simulink model "pmsmctrl"  (R2018a)
settings: Solver=FixedStepDiscrete  StartTime=0.0  StopTime=10.0  FixedStep=FastTsample / 10.  RelTol=1e-3  EnableMultiTasking=on
model workspace (MATLAB code in the model file):
  | cmdLim = Simulink.Parameter;
  | cmdLim.Value = 15;
  | cmdLim.Description = 'Limit for controlling the maximum surface command angle.';
  | cmdLim.Min = 0;
  | cmdLim.Max = 90;
  | cmdLim.DocUnits = 'deg';
  | 
  | dispGain = Simulink.Parameter;
  | dispGain.Value = 0.75;
  | dispGain.Description = 'Gain applied to the displacement error.';
  | dispGain.Min = 0;
  | dispGain.Max = [];
  | dispGain.DocUnits = 'deg/sec/deg';
  | 
  | dispLim = Simulink.Parameter;
  | dispLim.Value = 30;
  | dispLim.Description = 'Limit for controlling the maximum commanded angle.';
  | dispLim.Min = 0;
  | dispLim.Max = 180;
  | dispLim.DocUnits = 'deg';
  | 
  | intGain = Simulink.Parameter;
  | intGain.Value = 0.5;
  | intGain.Description = 'Gain applied to the integral error.';
  | intGain.Min = 0;
  | intGain.Max = [];
  | intGain.DocUnits = 'deg/sec/deg/sec';
  | 
  | intLim = Simulink.Parameter;
  | intLim.Value = 5;
  | intLim.Description = 'Limit for controlling the maximum commanded angle.';
  | intLim.Min = 0;
  | intLim.Max = 90;
  | intLim.DocUnits = 'deg';
  | 
  | rateGain = Simulink.Parameter;
  | rateGain.Value = 2;
  | rateGain.Description = 'Gain applied to the rate error.';
  | rateGain.Min = 0;
  | rateGain.Max = [];
  | rateGain.DocUnits = 'deg/deg/sec';
  | 
  | rateLim = Simulink.Parameter;
  | rateLim.Value = 6;
  | rateLim.Description = 'Limit for controlling the maximum commanded angle.';
  | rateLim.Min = 0;
  | rateLim.Max = 180;
  | rateLim.DocUnits = 'deg/sec';
  | 
  | hdgGain = Simulink.Parameter;
  | hdgGain.Value = 0.015;
undefined symbols (not defined in the file): MtrParams
libraries: powerlib_meascontrol x1
settings Model: RequirementInfo={} %GIDa_fe9045fd_0412_4b6e_8206_617cc20e6fde  FPTRunName=Active  Creator=elrobotista  LastModifiedBy=elrobotista
settings SolverCC: MinimalZcImpactIntegration=on
settings DataIOCC: SaveFormat=StructureWithTime  SaveOutput=off  SignalLogging=off  DSMLogging=off  SaveTime=off
settings OptimizationCC: DefaultParameterBehavior=Inlined  UseDivisionForNetSlopeComputation=on  UseFloatMulNetSlope=on  DefaultUnderspecifiedDataType=single  UseSpecifiedMinMax=on  InlineInvariantSignals=on  EnhancedBackFolding=on  PassReuseOutputArgsAs=Individual arguments  ZeroExternalMemoryAtStartup=off  ZeroInternalMemoryAtStartup=off  NoFixptDivByZeroProtection=on  EfficientFloat2IntCast=on  LifeSpan=1  OptimizeBlockOrder=speed  DifferentSizesBufferReuse=on  OptimizationCustomize=off  LabelGuidedReuse=on
settings DebuggingCC: AllowSymbolicDim=off  StrictBusMsg=ErrorOnBusTreatedAsVector  SFUnexpectedBacktrackingDiag=warning  SFNoUnconditionalDefaultTransitionDiag=warning  SFExecutionAtInitializationDiag=none
settings HardwareCC: ProdBitPerPointer=32  ProdBitPerSizeT=32  ProdBitPerPtrDiffT=32  ProdLargestAtomicInteger=Long  ProdLargestAtomicFloat=Double  ProdWordSize=32  ProdHWDeviceType=ARM Compatible->ARM Cortex
settings SFSimCC: MATLABDynamicMemAlloc=off
settings RTWCC: SystemTargetFile=ert.tlc  GenCodeOnly=on  PackageGeneratedCodeAndArtifacts=on  TemplateMakefile=ert_default_tmf  GenerateReport=on  BuildConfiguration=Faster Runs  IncludeHyperlinkInReport=on  LaunchReport=on  GenerateTraceInfo=on  GenerateTraceReport=on  GenerateTraceReportSl=on  GenerateTraceReportSf=on  GenerateTraceReportEml=on  GenerateCodeMetricsReport=on
settings CodeAppCC: ForceParamTrailComments=on  IgnoreCustomStorageClasses=off  OperatorAnnotations=on  SimulinkDataObjDesc=on  SFDataObjDesc=on  CustomSymbolStrGlobalVar=rt$N$M  CustomSymbolStrType=$N$M  CustomSymbolStrFcn=$N$M$F  CustomSymbolStrMacro=$N$M  InsertBlockDesc=on  EnableCustomComments=on  ReqsInCode=on
settings ERTTargetCC: TargetLangStandard=C99 (ISO)  MultiwordLength=2048  GenerateFullHeader=off  IncludeMdlTerminateFcn=off  SuppressErrorStatus=on  ERTCustomFileBanners=off  SupportAbsoluteTime=off  MultiInstanceERTCode=on  CodeInterfacePackaging=Reusable function  SupportNonFinite=off  SupportComplex=off  RemoveDisableFunc=on  InlinedParameterPlacement=NonHierarchical  MultiInstanceErrorCode=Warning  ERTCustomFileTemplate=example_file_process.tlc  ERTFilePackagingFormat=CompactWithDataFile
settings ConfigComp: CovScope=ReferencedModels  CovSaveName=covdata_rollAP  CovMetricSettings=dcmtrwe  CovHTMLOptions=-sRT=1 -aTS=1 -bRG=1 -bTC=1 -hTR=1 -nFC=0 -scm=1 -bcm=1 -xEv=0  CovSaveCumulativeToWorkspaceVar=on  CovSaveSingleToWorkspaceVar=on  CovCumulativeVarName=covCumulativeData_rollAP  CovReportOnPause=off  CovExternalEMLEnable=off  CovSFcnEnable=off

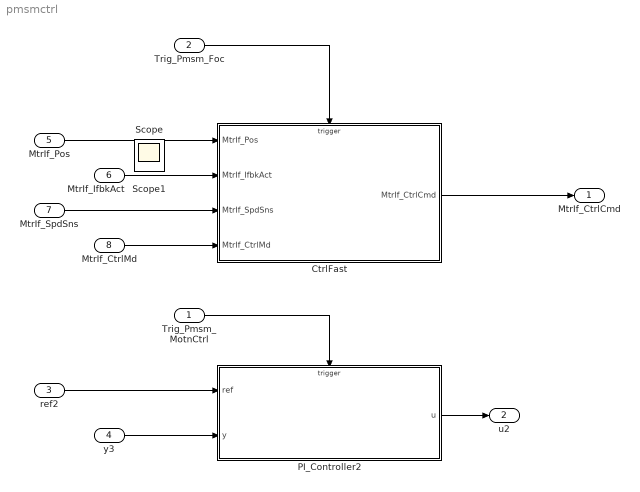
== system pmsmctrl ==
  Trig_Pmsm_MotnCtrl : Inport  OutDataTypeStr=double  OutputFunctionCall=on
  Trig_Pmsm_Foc : Inport  Port=2  OutDataTypeStr=double  OutputFunctionCall=on
  ref2 : Inport  Port=3
  y3 : Inport  Port=4
  MtrIf_Pos : Inport  Port=5
  MtrIf_IfbkAct : Inport  Port=6  PortDimensions=3
  MtrIf_SpdSns : Inport  Port=7
  MtrIf_CtrlMd : Inport  Port=8  OutDataTypeStr=Enum: MtrCtrlMd
  CtrlFast : Subsystem  TreatAsAtomicUnit=on  RTWFcnName=foo
  PI_Controller2 : Subsystem  TreatAsAtomicUnit=on  RTWFcnName=foo
  MtrIf_CtrlCmd : Outport
  u2 : Outport  Port=2
  Scope : Scope
  Scope1 : Scope
  wires:
  Trig_Pmsm_Foc/1 -> CtrlFast/Trigger
  Trig_Pmsm_MotnCtrl/1 -> PI_Controller2/Trigger
  PI_Controller2/1(u) -> u2/1
  ref2/1 -> PI_Controller2/1(ref)
  y3/1 -> PI_Controller2/2(y)
  MtrIf_Pos/1 -> CtrlFast/1(MtrIf_Pos)
  MtrIf_IfbkAct/1 -> CtrlFast/2(MtrIf_IfbkAct)
  MtrIf_CtrlMd/1 -> CtrlFast/4(MtrIf_CtrlMd)
  MtrIf_SpdSns/1 -> CtrlFast/3(MtrIf_SpdSns)
  CtrlFast/1(MtrIf_CtrlCmd) -> MtrIf_CtrlCmd/1

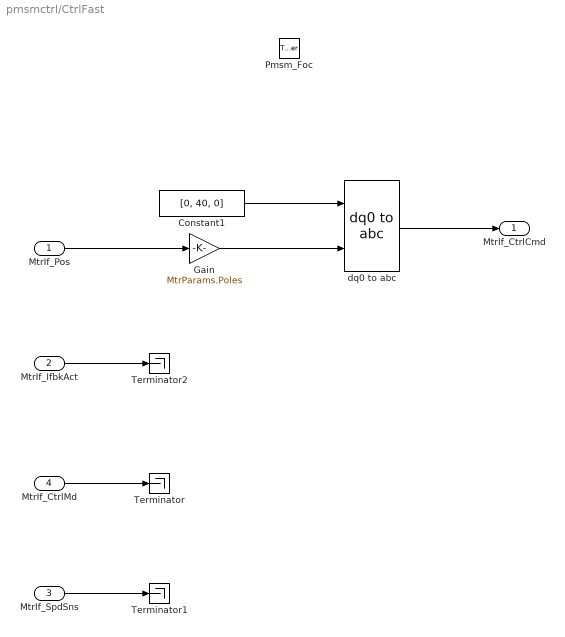
== system pmsmctrl/CtrlFast ==
  MtrIf_Pos : Inport
  MtrIf_IfbkAct : Inport  Port=2
  MtrIf_SpdSns : Inport  Port=3
  MtrIf_CtrlMd : Inport  Port=4  OutDataTypeStr=Enum: MtrCtrlMd
  Pmsm_Foc : TriggerPort  TriggerType=function-call  VariantControl=Variant  SampleTime=-1
  Constant1 : Constant  Value=[0, 40, 0]
  Gain : Gain  Gain=MtrParams.Poles
      settings: AttributesFormatString=%<Gain>
  Terminator : Terminator
  Terminator1 : Terminator
  Terminator2 : Terminator
  dq0 to abc : powerlib_meascontrol/Transformations/dq0 to abc  Alignment=90 degrees behind phase A axis
  MtrIf_CtrlCmd : Outport  InitialOutput=0
  wires:
  MtrIf_CtrlMd/1 -> Terminator/1
  MtrIf_SpdSns/1 -> Terminator1/1
  MtrIf_IfbkAct/1 -> Terminator2/1
  MtrIf_Pos/1 -> Gain/1
  dq0 to abc/1 -> MtrIf_CtrlCmd/1
  Constant1/1 -> dq0 to abc/1
  Gain/1 -> dq0 to abc/2

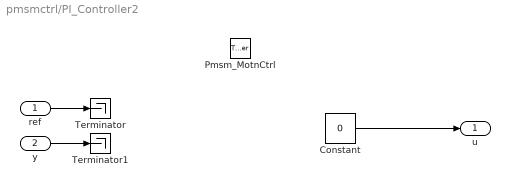
== system pmsmctrl/PI_Controller2 ==
  ref : Inport
  y : Inport  Port=2
  Pmsm_MotnCtrl : TriggerPort  TriggerType=function-call  VariantControl=Variant  SampleTime=-1
  Constant : Constant  Value=0  OutDataTypeStr=Inherit: Inherit via back propagation
  Terminator : Terminator
  Terminator1 : Terminator
  u : Outport  InitialOutput=0
  wires:
  y/1 -> Terminator1/1
  ref/1 -> Terminator/1
  Constant/1 -> u/1
